simulink model "ModeloControlePorPressaoRev5"  (R2014a)
settings: Solver=ode3  StartTime=0.0  StopTime=Tsimulacao  FixedStep=Tamostra  RelTol=1e-3
values from neighbouring files (symbols this model uses):
  Delay = 0.01    [CodigoTeste.m]    (also in CodigoTesteSimulador.m = 1.5; ControlePorPressaoRevFinal.m = input('Escolha o tempo para o delay do ventilador [s] '); PlotsDaSimulacaoFinal.m = 0.05; SimulacaoFinalDaPesquisa.m = ResultadosVentiladorInterrupcaoIntermitente(i,6))
  E = 38.1970    (= 38.197)    [CodigoTeste.m]    (also in CodigoTesteSimulador.m; ControlePorPressaoRevFinal.m = 50; PlotsDaSimulacaoFinal.m = 8.33333333333; SimulacaoFinalDaPesquisa.m = 1/ResultadosVentiladorInterrupcaoIntermitente(i,5))
  Habilitar = 0    [ControlePorPressaoRevFinal.m]    (also in PlotsDaSimulacaoFinal.m = 1; SimulacaoFinalDaPesquisa.m = 1)
  Hz = 1    [ControlePorPressaoRevFinal.m]    (also in PlotsDaSimulacaoFinal.m; SimulacaoFinalDaPesquisa.m = ResultadosVentiladorInterrupcaoIntermitente(i,10))
  Pasp = [-15.2979 -23.3827 -039.5964]    [CodigoTeste.m]    (also in CodigoTesteSimulador.m; ControlePorPressaoRevFinal.m = -200; PlotsDaSimulacaoFinal.m = -200; SimulacaoFinalDaPesquisa.m = -200)
  PressaoDelay = Pvent    (= 5)    [CodigoTeste.m]    (also in CodigoTesteSimulador.m; ControlePorPressaoRevFinal.m = 10; PlotsDaSimulacaoFinal.m = 10; SimulacaoFinalDaPesquisa.m = 10)
  Pvent = 5    [CodigoTeste.m]    (also in CodigoTesteSimulador.m; ControlePorPressaoRevFinal.m = 10; PlotsDaSimulacaoFinal.m = 10; SimulacaoFinalDaPesquisa.m = 10)
  Rrs = 3.3464    [CodigoTeste.m]    (also in CodigoTesteSimulador.m; ControlePorPressaoRevFinal.m = 5; PlotsDaSimulacaoFinal.m = 5; SimulacaoFinalDaPesquisa.m = ResultadosVentiladorInterrupcaoIntermitente(i,4))
  Tamanho_Sonda = 10    [CodigoTeste.m]    (also in CodigoTesteSimulador.m; ControlePorPressaoRevFinal.m = input('Qual o tamanho da sonda utilizada [FR]? 00, 06, 08, 1; PlotsDaSimulacaoFinal.m = 6; SimulacaoFinalDaPesquisa.m = ResultadosVentiladorInterrupcaoIntermitente(i,9))
  Tamostra = 0.001    [CodigoTeste.m]    (also in CodigoTesteSimulador.m; ControlePorPressaoRevFinal.m; PlotsDaSimulacaoFinal.m; SimulacaoFinalDaPesquisa.m)
  TOT = 7.5    [CodigoTeste.m]    (also in CodigoTesteSimulador.m; ControlePorPressaoRevFinal.m = input('Qual o tamanho do Tubo Orotraquial utilizado [mm]? 7.; PlotsDaSimulacaoFinal.m; SimulacaoFinalDaPesquisa.m = ResultadosVentiladorInterrupcaoIntermitente(i,8))
  VolumeInicial = VR+PressaoInicial/E    (= 0.130900332487)    [CodigoTeste.m]    (also in CodigoTesteSimulador.m; ControlePorPressaoRevFinal.m = 1.4; PlotsDaSimulacaoFinal.m = 2.4; SimulacaoFinalDaPesquisa.m = 2.4)
  VR = 0    [CodigoTeste.m]    (also in CodigoTesteSimulador.m; ControlePorPressaoRevFinal.m = 1.2; PlotsDaSimulacaoFinal.m = 1.2; SimulacaoFinalDaPesquisa.m = 1.2)
libraries: simulink x1
settings Model: Creator=Proprietário  LastModifiedBy=Texugão
settings DebuggingCC: MergeDetectMultiDrivingBlocksExec=error  FrameProcessingCompatibilityMsg=error

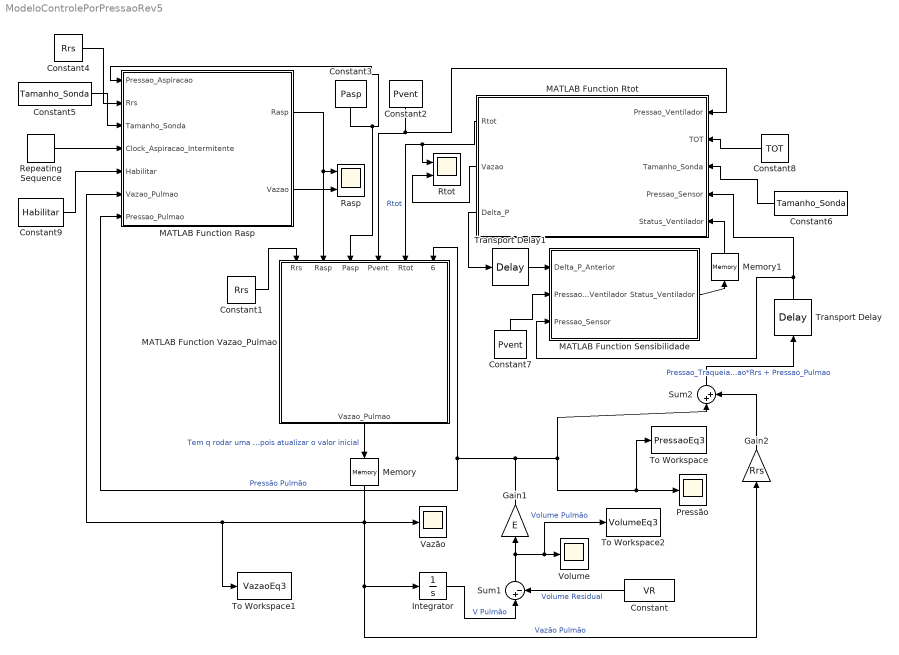
== system ModeloControlePorPressaoRev5 ==
  Constant : Constant  Value=VR
  Constant1 : Constant  Value=Rrs
  Constant2 : Constant  Value=Pvent
  Constant3 : Constant  Value=Pasp
  Constant4 : Constant  Value=Rrs
  Constant5 : Constant  Value=Tamanho_Sonda
  Constant6 : Constant  Value=Tamanho_Sonda
  Constant7 : Constant  Value=Pvent
  Constant8 : Constant  Value=TOT
  Constant9 : Constant  Value=Habilitar
  Gain1 : Gain  Gain=E
  Gain2 : Gain  Gain=Rrs
  Integrator : Integrator  InitialCondition=VolumeInicial
  MATLAB Function Rasp : MATLAB Function  TreatAsAtomicUnit=on
      settings: PermitHierarchicalResolution=ParametersOnly
  MATLAB Function Rtot : MATLAB Function  TreatAsAtomicUnit=on
      settings: PermitHierarchicalResolution=ParametersOnly
  MATLAB Function Sensibilidade : MATLAB Function  TreatAsAtomicUnit=on
      settings: PermitHierarchicalResolution=ParametersOnly
  MATLAB Function Vazao_Pulmao : MATLAB Function  TreatAsAtomicUnit=on
      settings: PermitHierarchicalResolution=ParametersOnly
  Memory : Memory
  Memory1 : Memory
  Pressão : Scope
      settings: TimeRange=auto  MaxDataPoints=5000  SaveToWorkspace=off  SaveName=PressaoPulmao  YMin=-0.77431  YMax=11.19715  SampleTime=-1  DataFormat=Array
  Rasp : Scope  NumInputPorts=2
      settings: TimeRange=auto  MaxDataPoints=5000  SaveName=ScopeData2  YMin=273.03119~0.49887  YMax=335.13281~0.65396  SampleTime=-1
  Repeating Sequence : simulink/Sources/Repeating Sequence  rep_seq_t=[0 1/Hz 1/Hz+0.001 2/Hz]  rep_seq_y=[1 1 0 0]
  Rtot : Scope  NumInputPorts=2
      settings: TimeRange=auto  MaxDataPoints=5000  YMin=-4.10485~-0.0804  YMax=36.94367~0.7236  SampleTime=-1
  Sum1 : Sum  Inputs=|+-
  Sum2 : Sum  Inputs=|++
  To Workspace : ToWorkspace  VariableName=PressaoEq3  SaveFormat=Timeseries  SampleTime=-1
  To Workspace1 : ToWorkspace  VariableName=VazaoEq3  SaveFormat=Timeseries  SampleTime=-1
  To Workspace2 : ToWorkspace  VariableName=VolumeEq3  SaveFormat=Timeseries  SampleTime=-1
  Transport Delay : TransportDelay  DelayTime=Delay  InitialOutput=PressaoDelay
  Transport Delay1 : TransportDelay  DelayTime=Tamostra
  Vazão : Scope
      settings: TimeRange=auto  MaxDataPoints=5000  SaveToWorkspace=off  SaveName=ScopeData2  YMin=-0.01146  YMax=-0.00769  SampleTime=-1  DataFormat=Array
  Volume : Scope
      settings: TimeRange=auto  MaxDataPoints=5000  SaveToWorkspace=off  SaveName=ScopeData3  YMin=1.19471  YMax=1.20059  SampleTime=-1  DataFormat=Array
  wires:
  Integrator/1 -> Sum1/1  "V Pulmão"
  Constant/1 -> Sum1/2  "Volume Residual"
  Memory/1 -> MATLAB Function Rasp/6(Vazao_Pulmao), To Workspace1/1, Integrator/1, Gain2/1, Vazão/1  "Vazão Pulmão"
  Sum1/1 -> To Workspace2/1, Volume/1, Gain1/1  "Volume Pulmão"
  Gain1/1 -> To Workspace/1, Pressão/1, Sum2/1, MATLAB Function Rasp/7(Pressao_Pulmao), MATLAB Function Vazao_Pulmao/6(Pressao_Pulmao)  "Pressão Pulmão"
  MATLAB Function Rasp/1(Rasp) -> MATLAB Function Vazao_Pulmao/2(Rasp), Rasp/1
  MATLAB Function Rtot/1(Rtot) -> Rtot/1, MATLAB Function Vazao_Pulmao/5(Rtot)  "Rtot"
  Constant2/1 -> MATLAB Function Rtot/1(Pressao_Ventilador), MATLAB Function Vazao_Pulmao/4(Pvent)
  MATLAB Function Vazao_Pulmao/1(Vazao_Pulmao) -> Memory/1  "Tem q rodar uma vez para  depois atualizar o valor inicial"
  Constant4/1 -> MATLAB Function Rasp/2(Rrs)
  Constant5/1 -> MATLAB Function Rasp/3(Tamanho_Sonda)
  Constant6/1 -> MATLAB Function Rtot/3(Tamanho_Sonda)
  Constant8/1 -> MATLAB Function Rtot/2(TOT)
  Constant1/1 -> MATLAB Function Vazao_Pulmao/1(Rrs)
  Constant3/1 -> MATLAB Function Vazao_Pulmao/3(Pasp), MATLAB Function Rasp/1(Pressao_Aspiracao)
  MATLAB Function Rasp/2(Vazao) -> Rasp/2
  MATLAB Function Rtot/2(Vazao) -> Rtot/2
  Repeating Sequence/1 -> MATLAB Function Rasp/4(Clock_Aspiracao_Intermitente)
  Constant9/1 -> MATLAB Function Rasp/5(Habilitar)
  Gain2/1 -> Sum2/2
  Sum2/1 -> Transport Delay/1  "Pressao_Traqueia = Vazao_Pulmao*Rrs + Pressao_Pulmao"
  Transport Delay/1 -> MATLAB Function Sensibilidade/3(Pressao_Sensor), MATLAB Function Rtot/4(Pressao_Sensor)
  MATLAB Function Rtot/3(Delta_P) -> Transport Delay1/1
  Transport Delay1/1 -> MATLAB Function Sensibilidade/1(Delta_P_Anterior)
  MATLAB Function Sensibilidade/1(Status_Ventilador) -> Memory1/1
  Memory1/1 -> MATLAB Function Rtot/5(Status_Ventilador)
  Constant7/1 -> MATLAB Function Sensibilidade/2(Pressao_Ventilador)

== matlab function ModeloControlePorPressaoRev5/MATLAB Function Sensibilidade ==
  data: Delta_P_Anterior input; Pressao_Ventilador input; Status_Ventilador output; Pressao_Sensor input
function Status_Ventilador = Sensibilidade_do_Ventilador(Delta_P_Anterior, Pressao_Ventilador, Pressao_Sensor)

Delta_P = abs(Pressao_Ventilador - Pressao_Sensor);

%Sensibilidade para o Sensor
%Somente ativa o ventilador caso a diferença de pressão seja maior que a sensibilidade
Sensibilidade = 0.9; %cmH2O
if Delta_P <= Sensibilidade %Não passou a sensibilidade?
    %Não passou da sensibilidade
    if Delta_P_Anterior < Delta_P %Delta_P está crescendo?
        %Sim. Para crescer, o ventilador tem que estar desligado
        Status_Ventilador = 0; 
    else
        %Não. Para diminuir, o ventilador tem que estar ligado
        Status_Ventilador = 1;
        if Delta_P == 0 %Chegou em 0?
            %Sim. Desliga o ventilador
            Status_Ventilador = 0;
        end
    end
else
    %Passou a sensibilidade
    Status_Ventilador = 1;
end

== matlab function ModeloControlePorPressaoRev5/MATLAB Function Rasp ==
  data: Pressao_Aspiracao input; Rrs input; Tamanho_Sonda input; Clock_Aspiracao_Intermitente input; Habilitar input; Vazao_Pulmao input; Rasp output; Pressao_Pulmao input; Vazao output
function [Rasp,Vazao] = Resistencia_da_Sonda_de_Aspiracao(Pressao_Aspiracao, Rrs, Tamanho_Sonda, Clock_Aspiracao_Intermitente,Habilitar, Vazao_Pulmao, Pressao_Pulmao)

%Equação de movimento para o sistema respiratório
Pressao_Traqueia = Vazao_Pulmao*Rrs + Pressao_Pulmao; 

Delta_P = abs(Pressao_Aspiracao - Pressao_Traqueia);

%Estimação da Vazão de acordo com o Tamanho da Sonda utilizada [00, 06, 08, 10, ou 12]
Vazao = 1;
Rasp = 1;
if Tamanho_Sonda == 0
    Vazao = 0;
elseif Tamanho_Sonda == 06
    Vazao = 0.001339*Delta_P^0.7939;   
elseif Tamanho_Sonda == 08
    Vazao = 0.01081*Delta_P^0.6338;
elseif Tamanho_Sonda == 10
    Vazao = 0.01501*Delta_P^0.6046;
elseif Tamanho_Sonda == 12
    Vazao = 0.03048*Delta_P^0.5689;
elseif Tamanho_Sonda == 14
    Vazao = 0.05087*Delta_P^0.5644;
end

%Aspiração Intermitente
if Habilitar == 1 %Permitiu
    if Clock_Aspiracao_Intermitente == 0 %Clock para parar de aspirar
        Vazao = 0; %Parou de aspirar
    end        
end


%Rasp
if Vazao == 0
    Rasp = 0;
else
    Rasp = Delta_P/Vazao;
end

== matlab function ModeloControlePorPressaoRev5/MATLAB Function Rtot ==
  data: Pressao_Ventilador input; TOT input; Tamanho_Sonda input; Pressao_Sensor input; Rtot output; Vazao output; Status_Ventilador input; Delta_P output
function [Rtot,Vazao,Delta_P] = Resistencia_do_TOT(Pressao_Ventilador, TOT, Tamanho_Sonda, Pressao_Sensor, Status_Ventilador)

%Equação de movimento para o sistema respiratório
% Pressao_Traqueia = Vazao_Pulmao*Rrs + Pressao_Pulmao;

Delta_P = abs(Pressao_Ventilador - Pressao_Sensor);

%Sensibilidade do Ventilador
if Status_Ventilador == 0
    Delta_P = 0;
end

% % % % % %Sensibilidade do Ventilador Beda
% % % % % persistent compensate; %ai a variavel compensate mantem o valor entre execuções
% % % % % if isempty(compensate)
% % % % %     compensate=false;
% % % % % end
% % % % % if Delta_P < 0.1 %threshold1 % tipo 0.1 cmh20
% % % % %     compensate = false;
% % % % % elseif Delta_P > 1 %threshold 2 %tipo 0.5-1 cmH20
% % % % %     compensate = true;
% % % % % end
% % % % % if compensate
% % % % %     %continua igual
% % % % % else
% % % % %     Delta_P =0;
% % % % % end 


    

%Estimação da Vazão de acordo com a combinação de TOT [7.5 ou 8.5] e Tamanho da Sonda utilizada [00, 06, 08, 10, ou 12]
Vazao = 1;
Rtot = 1;
if TOT == 7.5
    if Tamanho_Sonda == 0
        Vazao = 0.3833*Delta_P^0.5872;
    elseif Tamanho_Sonda == 06
        Vazao = 0.3223*Delta_P^0.5745;
    elseif Tamanho_Sonda == 08
        Vazao = 0.2745*Delta_P^0.5687;
    elseif Tamanho_Sonda == 10
        Vazao = 0.2682*Delta_P^0.5726;
    end
elseif TOT == 8.5
    if Tamanho_Sonda == 0
        Vazao = 0.548*Delta_P^0.5688;
    elseif Tamanho_Sonda == 06
        Vazao = 0.4413*Delta_P^0.5807;
    elseif Tamanho_Sonda == 08
        Vazao = 0.3795*Delta_P^0.5819;
    elseif Tamanho_Sonda == 10
        Vazao = 0.3808*Delta_P^0.5843;
    elseif Tamanho_Sonda == 12
        Vazao = 0.321*Delta_P^0.5871;
    end
end

if Vazao == 0
    Rtot = 0;
elseif Vazao > 0.5 %Vazão máxima do ventilador
    Vazao = 0.5;
    Rtot = Delta_P/Vazao;
else
    Rtot = Delta_P/Vazao;
end

== matlab function ModeloControlePorPressaoRev5/MATLAB Function Vazao_Pulmao ==
  data: Rrs input; Rasp input; Vazao_Pulmao output; Pasp input; Pvent input; Rtot input; Pressao_Pulmao input
function Vazao_Pulmao = Lei_de_Conservacao_da_Massa(Rrs, Rasp, Pasp, Pvent, Rtot, Pressao_Pulmao)

if Rasp == 0
    if Rtot == 0
        %Sistema em equilibrio -> V' = -E(V-VR)/Rrs
        Vazao_Pulmao = 0;
    else
        %Sem circuito de aspiração -> V' = (Pvent/Rtot -E(V-VR)/Rtot)/(1+(Rrs/Rtot))
        Vazao_Pulmao = (Pvent/Rtot - Pressao_Pulmao*(1/Rtot))/(1+(Rrs/Rtot));
    end
    
elseif Rtot == 0
    %Diferença entre delta_P do Pulmão e Ventilador = 0 -> V' = (Pasp/Rasp -E(V-VR)/Rasp)/(1+(Rrs/Rasp))
    Vazao_Pulmao = (Pasp/Rasp - Pressao_Pulmao*(1/Rasp))/(1+(Rrs/Rasp));
else
    %Funcionamento Normal
    Vazao_Pulmao = (Pasp/Rasp + Pvent/Rtot - Pressao_Pulmao*(1/Rasp+1/Rtot))/(1+(1/Rtot+1/Rasp)*Rrs);
end
